simulink subsystem "HMT_Controller"  (R2022b)
settings: Solver=VariableStepAuto  StartTime=0.0  StopTime=10.0  RelTol=1e-3
libraries: simulink x1
settings Model: Creator=david

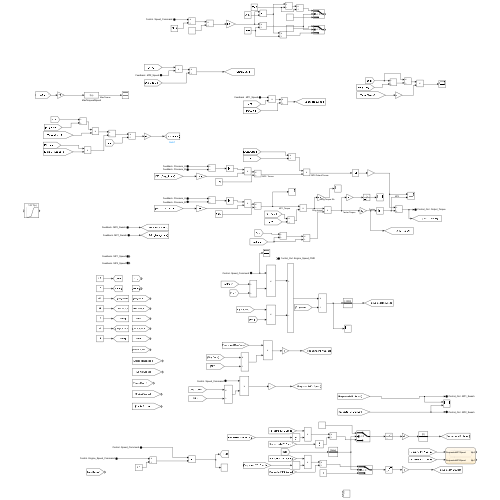
[thumbnail: Simulink's stored preview of the top-level diagram]
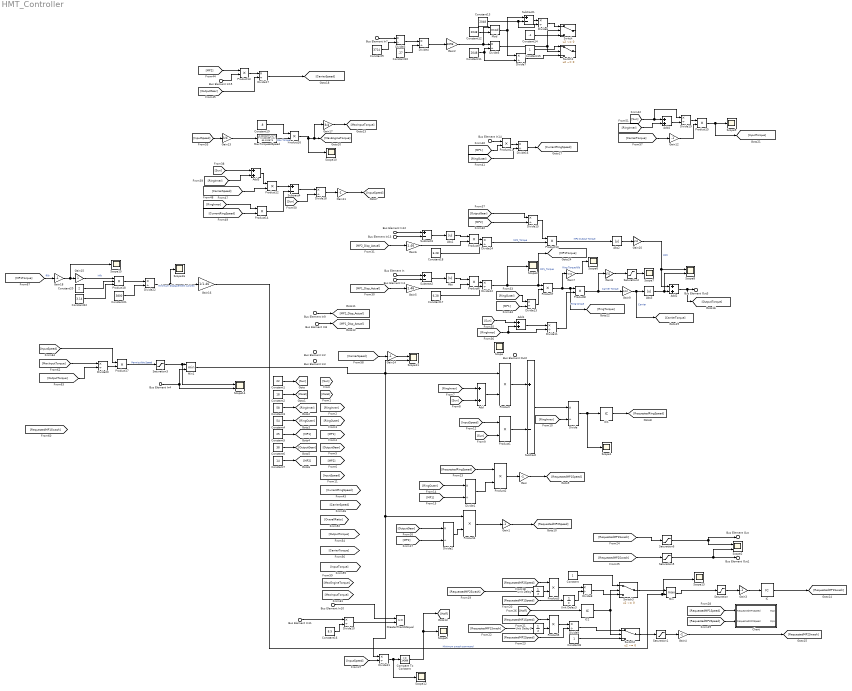
== system HMT_Controller ==
  Bus Element In : Inport  PortName=Feedback  Element=Pressure_A
  Bus Element In12 : Inport  PortName=Feedback  Element=Pressure_A
  Bus Element In1 : Inport  PortName=Feedback  Element=Pressure_B
  Bus Element In13 : Inport  PortName=Feedback  Element=Pressure_B
  Bus Element In2 : Inport  PortName=Feedback  Element=MP1_Speed
  Bus Element In14 : Inport  PortName=Feedback  Element=MP1_Speed
  Bus Element In3 : Inport  PortName=Feedback  Element=MP2_Speed
  Bus Element In15 : Inport  PortName=Feedback  Element=MP2_Speed
  Bus Element In8 : Inport  PortName=Feedback  Element=MP1_Swash
  Bus Element In9 : Inport  PortName=Feedback  Element=MP2_Swash
  Bus Element In4 : Inport  Port=2  PortName=Control  Element=Speed_Command
  Bus Element In7 : Inport  Port=2  PortName=Control  Element=Speed_Command
  Bus Element In10 : Inport  Port=2  PortName=Control  Element=Speed_Command
  Bus Element In11 : Inport  Port=2  PortName=Control  Element=Engine_Speed_Command
  Abs{,1..3} (4 alike) : Abs  SaturateOnIntegerOverflow=off
  Add{,1..4} (5 alike) : Sum
  Chart : Stateflow chart  TreatAsAtomicUnit=on
  Compare To Constant : simulink/Logic and Bit Operations/Compare To Constant  relop=>=  const=.14389  OutDataTypeStr=boolean
  Constant : Constant
  Constant1 : Constant  Value=22
  Constant10 : Constant  Value=.27
  Constant11 : Constant  Value=2048
  Constant12 : Constant  Value=2048
  Constant13 : Constant  Value=2048
  Constant14 : Constant  Value=-1
  Constant15 : Constant
  Constant16 : Constant  Value=8.5
  Constant17 : Constant  Value=6.28
  Constant18 : Constant  Value=6.28
  Constant19 : Constant  Value=.8
  Constant2 : Constant  Value=18
  Constant20 : Constant  Value=2
  Constant21 : Constant  Value=3800
  Constant22 : Constant  Value=3.14
  Constant3 : Constant  Value=58
  Constant4 : Constant  Value=54
  Constant5 : Constant  Value=25
  Constant6 : Constant  Value=38
  Constant7 : Constant  Value=14
  Constant8 : Constant
  Constant9 : Constant  Value=3724
  Divide{,1..22} (23 alike) : Product  Inputs=*/
  Gain{,1,3..4,11..12,14,18} (8 alike) : Gain  Gain=-1
  Gain10 : Gain  Gain=1/12
  Gain13 : Gain  Gain=3/4
  Gain15 : Gain
  Gain16 : Gain  Gain=1/1.46
  Gain17 : Gain  Gain=3/4
  Gain2 : Gain  Gain=4096
  Gain5 : Gain  Gain=1.46
  Gain6 : Gain  Gain=1.46
  Gain7 : Gain  Gain=-1/12
  Gain8 : Gain  Gain=1/12
  Gain9 : Gain  Gain=1/12
  GreaterThanOrEqual : RelationalOperator  OutDataTypeStr=boolean  RndMeth=Simplest  InputSameDT=off
  IC : InitialCondition  Value=0
  IC1 : InitialCondition  Value=-1000
  IC2 : InitialCondition  Value=false
  MaxTorqueatSpeed : Fcn  Expr=-0.000019*u(1)^2 + 0.102035*u(1) - 80.132873
  Min : MinMax  Function=max  Inputs=2
  Min1 : MinMax  Inputs=2
  Mod : Math  Operator=mod
  Product{,1..17} (18 alike) : Product
  Product18 : Product  Inputs=3
  Saturation : Saturate  UpperLimit=1  LowerLimit=0
  Saturation1 : Saturate  UpperLimit=1  LowerLimit=-1
  Saturation2 : Saturate  UpperLimit=1000  LowerLimit=-1000
  Saturation3 : Saturate  UpperLimit=2000  LowerLimit=0
  Saturation5 : Saturate  UpperLimit=1  LowerLimit=-1
  Saturation6 : Saturate  UpperLimit=1  LowerLimit=-1
  Scope{,1,3,5..7,9..10,12,15..16} (11 alike) : Scope
  Scope{2,8,11,13..14} (5 alike) : Scope  NumInputPorts=2
  Subtract{,1..4} (5 alike) : Sum  Inputs=+-
  Switch : Switch  Criteria=u2 ~= 0  SaturateOnIntegerOverflow=off  InputSameDT=off
  Switch1 : Switch  Criteria=u2 ~= 0  SaturateOnIntegerOverflow=off  InputSameDT=off
  Switch2 : Switch  Criteria=u2 ~= 0  Threshold=688  SaturateOnIntegerOverflow=off  InputSameDT=off
  Switch3 : Switch  Criteria=u2 ~= 0  Threshold=688  SaturateOnIntegerOverflow=off  InputSameDT=off
  Unit Delay : UnitDelay  InitialCondition=1  SampleTime=-1  HasFrameUpgradeWarning=on
  Unit Delay1 : UnitDelay  SampleTime=-1  HasFrameUpgradeWarning=on
  Unit Delay3 : UnitDelay  InitialCondition=1  SampleTime=-1  HasFrameUpgradeWarning=on
  Bus Element Out : Outport  VectorParamsAs1DForOutWhenUnconnected=off  PortName=Control_Out  Element=MP1_Swash
  Bus Element Out1 : Outport  VectorParamsAs1DForOutWhenUnconnected=off  PortName=Control_Out  Element=MP2_Swash
  Bus Element Out2 : Outport  VectorParamsAs1DForOutWhenUnconnected=off  PortName=Control_Out  Element=Engine_Speed_CMD
  Bus Element Out3 : Outport  VectorParamsAs1DForOutWhenUnconnected=off  PortName=Control_Out  Element=Output_Torque
  wires:
  Constant1/1 -> [Sun]
  Constant2/1 -> [Planet]
  Constant4/1 -> [RingOuter]
  Constant3/1 -> [RingInner]
  Constant5/1 -> [MP1]
  Constant6/1 -> [OutputGear]
  Constant7/1 -> [MP2]
  [RingInner] -> Add/1
  [Sun] -> Add/2
  Add/1 -> Product/2
  [Sun] -> Product1/2
  Product1/1 -> Subtract/2
  Product/1 -> Subtract/1
  Subtract/1 -> Divide/1
  [RingInner] -> Divide/2
  [InputSpeed] -> Product1/1
  Divide/1 -> IC1/1, Scope1/1
  [RequestedRingSpeed] -> Product2/1
  [RingOuter] -> Divide1/1
  [MP1] -> Divide1/2
  Divide1/1 -> Product2/2
  Product2/1 -> Gain/1
  Gain/1 -> [RequestedMP1Speed]
  Divide2/1 -> Product4/2
  [OutputGear] -> Divide2/1
  [MP2] -> Divide2/2
  Gain1/1 -> [RequestedMP2Speed]
  Bus Element In7/1 -> Divide3/1
  Constant9/1 -> Divide3/2
  Constant10/1 -> Divide4/2
  Divide3/1 -> Divide4/1
  Divide4/1 -> Gain2/1
  Gain2/1 -> Mod/1, Divide5/1
  Constant11/1 -> Divide7/2, Divide5/2
  Constant12/1 -> Mod/2
  Constant13/1 -> Divide6/2, Subtract1/2
  Subtract1/1 -> Divide6/1
  Divide6/1 -> Switch/1
  Constant14/1 -> Switch/3
  Divide5/1 -> Switch/2, Switch1/2
  Constant15/1 -> Switch1/1
  Mod/1 -> Subtract1/1, Divide7/1
  Divide7/1 -> Switch1/3
  [RequestedMP2Speed] -> Product3/1
  [RequestedMP1Speed] -> Unit Delay3/1
  [RequestedMP2Speed] -> Divide9/2
  Product5/1 -> Divide9/1
  [RequestedMP1Swash] -> Unit Delay1/1
  [RequestedMP1Speed] -> Product5/1
  Switch2/1 -> Saturation1/1
  Unit Delay/1 -> Product3/2
  Unit Delay1/1 -> Product5/2
  Constant/1 -> Switch3/1
  Divide8/1 -> Switch3/3
  Bus Element In9/1 -> [MP2_Disp_Actual]
  Bus Element In8/1 -> [MP1_Disp_Actual]
  Divide9/1 -> Switch2/1
  Constant8/1 -> Switch2/3
  [RequestedMP2Swash] -> Unit Delay/1
  Product3/1 -> Divide8/1
  Unit Delay3/1 -> Divide8/2
  Saturation/1 -> Gain3/1
  Gain3/1 -> IC/1
  Saturation1/1 -> Gain4/1
  IC1/1 -> [RequestedRingSpeed]
  [RequestedMP1Swash] -> Saturation6/1
  IC2/1 -> Switch2/2, Switch3/2
  [RequestedMP1Speed] -> Chart/1(RequestedMP1Speed)
  [RequestedMP2Speed] -> Chart/2(RequestedMP2Speed)
  [Half] -> IC2/1
  Gain4/1 -> [RequestedMP2Swash]
  Constant16/1 -> Divide10/2
  Bus Element In10/1 -> GreaterThanOrEqual/1
  Divide10/1 -> GreaterThanOrEqual/2
  Bus Element In11/1 -> Divide10/1
  Bus Element In/1 -> Subtract2/1
  Bus Element In1/1 -> Subtract2/2
  Subtract2/1 -> Abs/1
  Abs/1 -> Product6/1
  [MP1_Disp_Actual] -> Gain5/1
  Add1/1 -> Divide11/1
  Gain5/1 -> Product6/2
  Product6/1 -> Divide12/1
  Constant17/1 -> Divide12/2
  Product8/1 -> Gain8/1, Gain9/1  "Carrier Torque"
  Divide12/1 -> Product7/1, [MP1Torque], Scope3/1  "MP1_Torque"
  Divide13/1 -> Product7/2
  Product7/1 -> Product8/1, [RingTorque], Gain7/1  "Ring torque"
  Divide11/1 -> Product8/2
  Gain7/1 -> Scope6/1  "Ring Torque ftlb"
  [MP1] -> Divide13/2
  [RingOuter] -> Divide13/1
  Saturation2/1 -> Scope7/1
  Gain8/1 -> Saturation2/1
  [Sun] -> Add1/1
  [RingInner] -> Add1/2, Divide11/2
  Constant18/1 -> Divide14/2
  Product9/1 -> Divide14/1
  Gain6/1 -> Product9/2
  [MP2_Disp_Actual] -> Gain6/1
  Abs1/1 -> Product9/1
  Subtract3/1 -> Abs1/1
  Bus Element In13/1 -> Subtract3/2
  Bus Element In12/1 -> Subtract3/1
  Divide14/1 -> Product10/2  "MP2_Torque"
  [OutputGear] -> Divide15/1
  [MP2] -> Divide15/2
  Divide15/1 -> Product10/1
  Gain9/1 -> [CarrierTorque], Abs3/1  "Carrier"
  Product10/1 -> Abs2/1  "MP2 Output Torque"
  Gain10/1 -> Add2/1, Scope8/1  "MP2"
  Abs2/1 -> Gain10/1
  Add2/1 -> Bus Element Out3/1, [OutputTorque]
  Bus Element In14/1 -> Product11/1
  [MP1] -> Product11/2
  Product11/1 -> Divide16/1
  [RingOuter] -> Divide16/2
  Divide16/1 -> [CurrentRingSpeed]
  [Sun] -> Add3/1
  [RingInner] -> Add3/2
  Add3/1 -> Product12/1
  [MP2] -> Product13/1
  Bus Element In15/1 -> Product13/2
  Product13/1 -> Divide17/1
  [OutputGear] -> Divide17/2
  [CarrierSpeed] -> Product12/2
  [CurrentRingSpeed] -> Product14/2
  [RingInner] -> Product14/1
  Product12/1 -> Subtract4/1
  Product14/1 -> Subtract4/2
  Subtract4/1 -> Divide18/1
  [Sun] -> Divide18/2
  Divide18/1 -> Gain11/1
  Gain11/1 -> [InputSpeed]
  Divide17/1 -> [CarrierSpeed]
  Add4/1 -> Divide19/2
  [RingInner] -> Add4/2
  [Sun] -> Add4/1, Divide19/1
  Abs3/1 -> Add2/2, Scope8/2
  Divide19/1 -> Product15/1
  [CarrierTorque] -> Gain12/1
  Product15/1 -> Scope9/1, [InputTorque]
  Gain12/1 -> Product15/2
  [InputSpeed] -> Gain13/1
  Gain13/1 -> MaxTorqueatSpeed/1
  Product16/1 -> [MaxEngineTorque], Gain17/1, Scope10/1
  MaxTorqueatSpeed/1 -> Product16/2  "Max Torque"
  Constant19/1 -> Product16/1
  Gain17/1 -> [MaxInputTorque]
  [MaxInputTorque] -> Divide20/1
  [OutputTorque] -> Divide20/2
  Divide20/1 -> Product17/2
  [InputSpeed] -> Product17/1
  Product17/1 -> Saturation3/1  "Permissible Speed"
  Bus Element In4/1 -> Min1/2, Scope14/2
  [CarrierSpeed] -> Gain14/1
  Gain14/1 -> Scope11/1
  Product4/1 -> Gain1/1
  [InputSpeed] -> Divide21/2
  Min1/1 -> Product/1, Product4/1, Divide21/1, Scope11/2
  Divide21/1 -> Compare To Constant/1, Scope12/1
  Compare To Constant/1 -> [Half], Scope5/1
  Saturation3/1 -> Scope14/1, Min1/1
  IC/1 -> [RequestedMP1Swash]
  [RequestedMP2Swash] -> Saturation5/1
  [MP1Torque] -> Gain18/1  "ftlb"
  Gain15/1 -> Product18/1  "inlb"
  Constant20/1 -> Product18/2
  Constant22/1 -> Product18/3
  Product18/1 -> Divide22/1
  Constant21/1 -> Divide22/2
  Divide22/1 -> Scope16/1, Gain16/1  "Minimum displacement cuin/rev"
  Gain16/1 -> Min/2, Scope13/2  "Minimum swash command"
  Gain18/1 -> Gain15/1, Scope15/1
  Switch3/1 -> Min/1
  Min/1 -> Saturation/1
  Saturation5/1 -> Bus Element Out1/1, Scope2/2
  Saturation6/1 -> Scope2/1, Bus Element Out/1

== stateflow chart HMT_Controller/Chart ==
  state phase_one
    en:
    Mp1=0;
    Mp2=-1;
    du:
    Mp2=-1;
    Mp1=(RequestedMP2Speed*Mp2)/RequestedMP1Speed;
  state phase_two
    en,du:
    Mp1=-1;
    Mp1=(RequestedMP1Speed*Mp1)/RequestedMP2Speed;
  (default) -> phase_one
  phase_one -> phase_two : [Mp1>=1]
  data: RequestedMP1Speed input; RequestedMP2Speed input; Mp2 output; Mp1 output
